simulink model "simu_afbs_for_publish"  (Simulink 9.3)
settings: Solver=FixedStepAuto  StartTime=0.0  StopTime=simu.time  FixedStep=1e-5  RelTol=1e-4  EnableMultiTasking=on
values from neighbouring files (symbols this model uses):
  sys = tf(sys_zpk)    [main.m]    (also in main_compare_single_dual.m; main_cost_space.m; myFitness.m; myFitness_lamba_u.m)
undefined symbols (not defined in the file): simu
settings Model: Creator=Xiaotian  LastModifiedBy=Steven
settings DataIOCC: LimitDataPoints=on  SignalLoggingSaveFormat=Dataset
settings DebuggingCC: UnderspecifiedInitializationDetection=Simplified  MergeDetectMultiDrivingBlocksExec=error  FcnCallInpInsideContextMsg=error
settings GRTTargetCC: GeneratePreprocessorConditionals=Disable all  CombineOutputUpdateFcns=on  GRTInterface=off

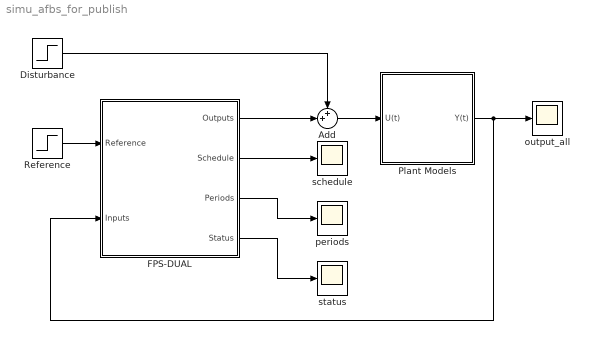
== system simu_afbs_for_publish ==
  Add : Sum  Inputs=++|
  Disturbance : Step  Time=0  After=0  SampleTime=0
  FPS-DUAL : Subsystem  mask{afbs_params__=simu.afbs_params, task_params__=simu.taskset}
      mask prompts: afbs_params__ "AFBS_Parameters"; task_params__ "Taskset"
      mask DialogControl DescTextVar Prompt: A Fixed-Priority Scheduler that supports adaptive and flexible scheduling.
  Plant Models : Subsystem
  Reference : Step  Time=0  SampleTime=0
  output_all : Scope
  periods : Scope
  schedule : Scope
  status : Scope
  wires:
  FPS-DUAL/2(Schedule) -> schedule/1
  Plant Models/1(Y(t)) -> output_all/1, FPS-DUAL/2(Inputs)
  FPS-DUAL/3(Periods) -> periods/1
  Reference/1 -> FPS-DUAL/1(Reference)
  Disturbance/1 -> Add/1
  FPS-DUAL/1(Outputs) -> Add/2
  Add/1 -> Plant Models/1(U(t))
  FPS-DUAL/4(Status) -> status/1

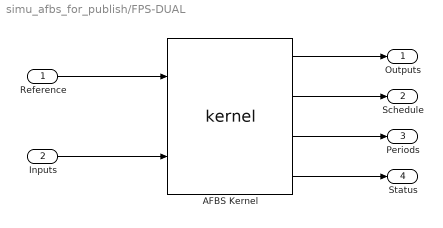
== system simu_afbs_for_publish/FPS-DUAL ==
  Reference : Inport
  Inputs : Inport  Port=2
  AFBS Kernel : S-Function  FunctionName=kernel  Parameters=afbs_params__,task_params__  SFunctionDeploymentMode=off  EnableBusSupport=off
  Outputs : Outport
  Schedule : Outport  Port=2
  Periods : Outport  Port=3
  Status : Outport  Port=4
  wires:
  AFBS Kernel/1 -> Outputs/1
  AFBS Kernel/2 -> Schedule/1
  AFBS Kernel/3 -> Periods/1
  Reference/1 -> AFBS Kernel/1
  Inputs/1 -> AFBS Kernel/2
  AFBS Kernel/4 -> Status/1

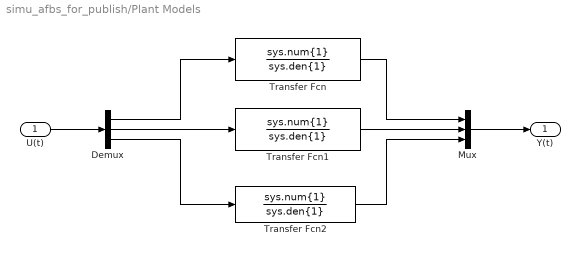
== system simu_afbs_for_publish/Plant Models ==
  U(t) : Inport
  Demux : Demux  Outputs=3
  Mux : Mux  Inputs=3
  Transfer Fcn : TransferFcn  Numerator=sys.num{1}  Denominator=sys.den{1}
  Transfer Fcn1 : TransferFcn  Numerator=sys.num{1}  Denominator=sys.den{1}
  Transfer Fcn2 : TransferFcn  Numerator=sys.num{1}  Denominator=sys.den{1}
  Y(t) : Outport
  wires:
  U(t)/1 -> Demux/1
  Demux/1 -> Transfer Fcn/1
  Demux/2 -> Transfer Fcn1/1
  Demux/3 -> Transfer Fcn2/1
  Transfer Fcn/1 -> Mux/1
  Transfer Fcn1/1 -> Mux/2
  Transfer Fcn2/1 -> Mux/3
  Mux/1 -> Y(t)/1
